simulink model "gimbal_nonlinear"  (R2019b)
settings: Solver=VariableStepAuto  StartTime=0.0  StopTime=200  RelTol=1e-3
values from neighbouring files (symbols this model uses):
  Fe = ones(length(phi),1)*(m*g)    [main_rocketmodel.m]    (also in main_sim_rocket.m = thrust_eq+(2e6)*square(t_signal,25); rocket_model.m = ones(1000,1)*(300); sim_lin.m = ones(length(phi),1)*(2*10^6))
  Fs = Fl-Fr    [main_rocketmodel.m]    (also in main_sim_rocket.m; rocket_model.m)
  g = 9.8    [main_rocketmodel.m]    (also in main_sim_rocket.m; rocket_model.m; sim_lin.m; test_bangbang.m)
  J_T = 40267    [main_rocketmodel.m]    (also in main_sim_rocket.m; rocket_model.m = 10)
  lower_body = l1+ln    (= 15)    [rocket_model.m]
  m = 549054    [main_rocketmodel.m]    (also in main_sim_rocket.m; rocket_model.m = 25.4; sim_lin.m; test_bangbang.m)
  theta = 0    [main_rocketmodel.m]    (also in main_sim_rocket.m; rocket_model.m)
  upper_body = l2    (= 3)    [rocket_model.m]
settings Model: Creator=bia  LastModifiedBy=bia
settings DataIOCC: ExternalInput=[t, phi]  LoadExternalInput=on

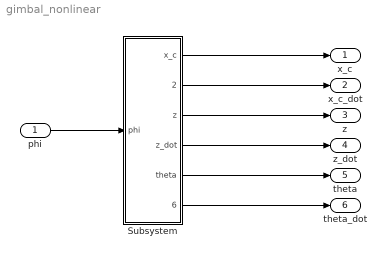
== system gimbal_nonlinear ==
  phi : Inport
  Subsystem : Subsystem
  x_c : Outport
  x_c_dot : Outport  Port=2
  z : Outport  Port=3
  "z_dot " : Outport  Port=4
  theta : Outport  Port=5
  "theta_dot " : Outport  Port=6
  wires:
  Subsystem/4("z_dot ") -> "z_dot "/1
  Subsystem/6("theta_dot ") -> "theta_dot "/1
  Subsystem/2(x_c_dot) -> x_c_dot/1
  Subsystem/5(theta) -> theta/1
  Subsystem/3(z) -> z/1
  phi/1 -> Subsystem/1(phi)
  Subsystem/1(x_c) -> x_c/1

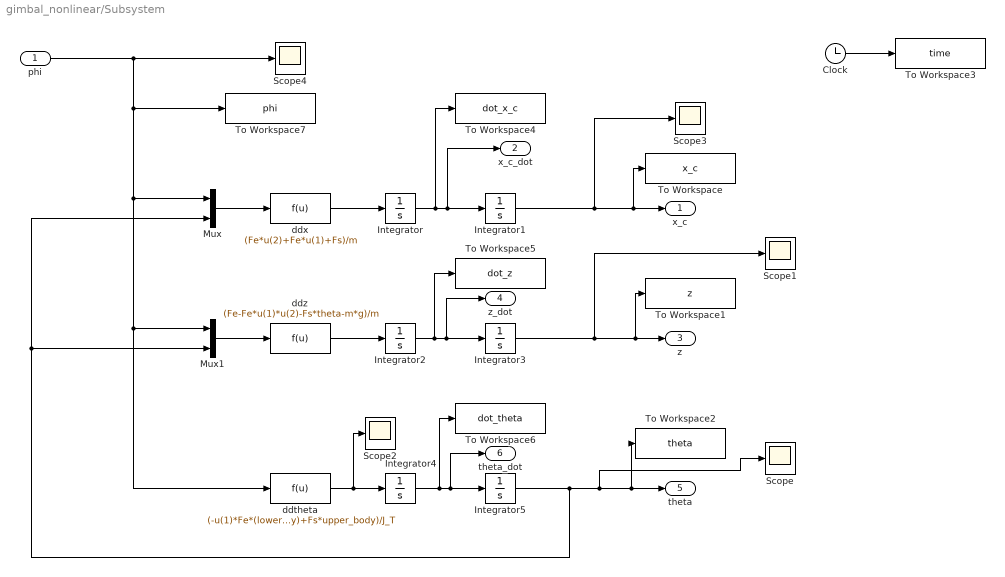
== system gimbal_nonlinear/Subsystem ==
  phi : Inport
  Clock : Clock
  Integrator : Integrator  ContinuousStateAttributes='x_c_dot'
  Integrator1 : Integrator  ContinuousStateAttributes='x_c'
  Integrator2 : Integrator  ContinuousStateAttributes='z_dot'
  Integrator3 : Integrator  ContinuousStateAttributes='z'
  Integrator4 : Integrator  ContinuousStateAttributes='theta_dot'
  Integrator5 : Integrator
  Mux : Mux  Inputs=2
  Mux1 : Mux  Inputs=2
  Scope{,1..4} (5 alike) : Scope
  To Workspace : ToWorkspace  VariableName=x_c  SaveFormat=Timeseries  SampleTime=-1
  To Workspace1 : ToWorkspace  VariableName=z  SaveFormat=Timeseries  SampleTime=-1
  To Workspace2 : ToWorkspace  VariableName=theta  SaveFormat=Timeseries  SampleTime=-1
  To Workspace3 : ToWorkspace  VariableName=time  SaveFormat=Timeseries  SampleTime=-1
  To Workspace4 : ToWorkspace  VariableName=dot_x_c  SaveFormat=Timeseries  SampleTime=-1
  To Workspace5 : ToWorkspace  VariableName=dot_z  SaveFormat=Timeseries  SampleTime=-1
  To Workspace6 : ToWorkspace  VariableName=dot_theta  SaveFormat=Timeseries  SampleTime=-1
  To Workspace7 : ToWorkspace  VariableName=phi  SaveFormat=Timeseries  SampleTime=-1
  "ddtheta " : Fcn  Expr=(-u(1)*Fe*(lower_body)+Fs*upper_body)/J_T
  ddx : Fcn  Expr=(Fe*u(2)+Fe*u(1)+Fs)/m
  ddz : Fcn  Expr=(Fe-Fe*u(1)*u(2)-Fs*theta-m*g)/m
  x_c : Outport
  x_c_dot : Outport  Port=2
  z : Outport  Port=3
  "z_dot " : Outport  Port=4
  theta : Outport  Port=5
  "theta_dot " : Outport  Port=6
  wires:
  ddx/1 -> Integrator/1
  ddz/1 -> Integrator2/1
  Integrator1/1 -> To Workspace/1, x_c/1, Scope3/1
  Integrator2/1 -> To Workspace5/1, "z_dot "/1, Integrator3/1
  "ddtheta "/1 -> Scope2/1, Integrator4/1
  Integrator4/1 -> To Workspace6/1, "theta_dot "/1, Integrator5/1
  Integrator3/1 -> To Workspace1/1, z/1, Scope1/1
  Integrator5/1 -> Scope/1, To Workspace2/1, theta/1, Mux1/2, Mux/2
  Mux/1 -> ddx/1
  Mux1/1 -> ddz/1
  phi/1 -> To Workspace7/1, Mux1/1, "ddtheta "/1, Mux/1, Scope4/1
  Clock/1 -> To Workspace3/1
  Integrator/1 -> Integrator1/1, x_c_dot/1, To Workspace4/1
